simulink model "jiangyong_ZB2305010116"  (R2022b)
settings: Solver=VariableStepAuto  StartTime=0.0  StopTime=5  RelTol=1e-3
libraries: commdigbbndpm3 x4, commchan3 x2, commsink2 x2, commrandsrc3 x2
settings Model: Creator=JY  LastModifiedBy=JY

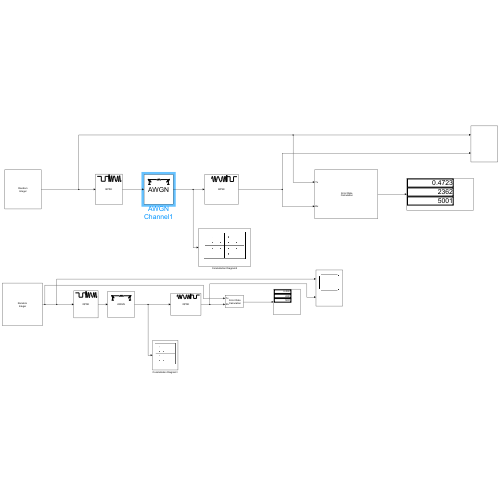
[thumbnail: Simulink's stored preview of the top-level diagram]
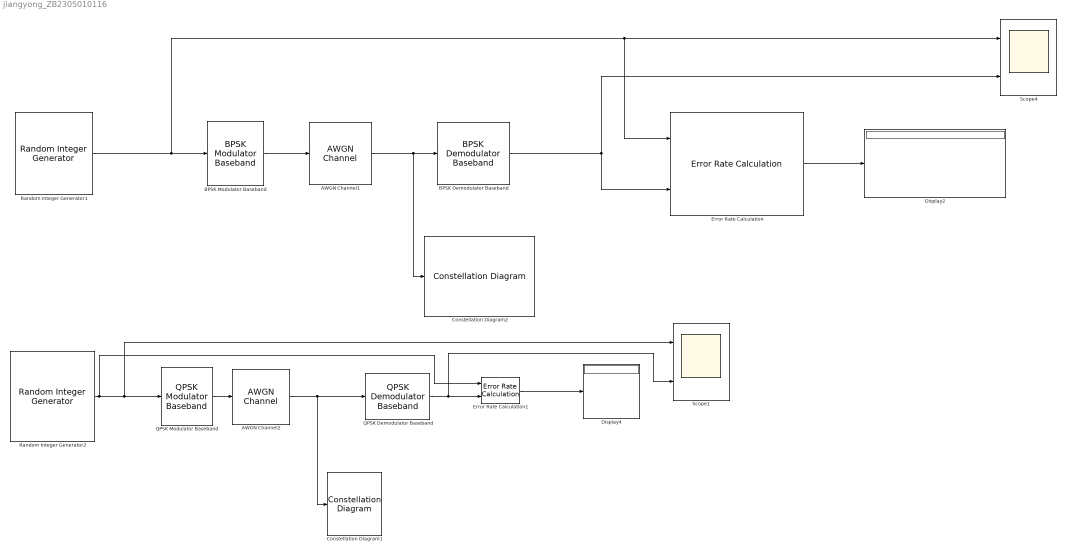
== system jiangyong_ZB2305010116 ==
  AWGN Channel1 : commchan3/AWGN Channel  InputProcessing=Columns as channels (frame based)  seed=67  noiseMode="Signal to noise ratio  (Eb/No)"  EbNodB=1  EsNodB=50  SNRdB=0  bitsPerSym=1  Ps=1  Tsym=1  variance=1
  AWGN Channel2 : commchan3/AWGN Channel  InputProcessing=Columns as channels (frame based)  seed=67  noiseMode="Signal to noise ratio  (Eb/No)"  EbNodB=9  EsNodB=10  SNRdB=0  bitsPerSym=1  Ps=2  Tsym=0.01  variance=1
  BPSK Demodulator Baseband : commdigbbndpm3/BPSK Demodulator Baseband  DecType=Hard decision  VarSource=Dialog  Variance=1  Ph=0  outDtype=Inherit via internal rule  derotateFactorWordLen=16  derotateFactorDataTypeStr=Inherit: Same word length as input  derotateFactorLastDataTypeStr=Inherit: Same word length as input
  BPSK Modulator Baseband : commdigbbndpm3/BPSK Modulator Baseband  Ph=0  outDtype=double  outWordLen=16  outUDDataType=sfix(16)  outFracLenMode=Best precision  outFracLen=15  outDataTypeStr=double  outLastDataTypeStr=double
  Constellation Diagram1 : ConstellationDiagram  WindowPosition=[707.000000,41.000000,600.000000,600.000000,]  ScopeFrameLocation=window  SymbolsToDisplaySource=Property  SymbolsToDisplay=1000  ReferenceConstellation=QPSK  XLimits=[-1.46,1.46]  YLimits=[-1.38,1.38]
  Constellation Diagram2 : ConstellationDiagram  WindowPosition=[-107.000000,-37.000000,1536.000000,793.000000,]  ScopeFrameLocation=window  SymbolsToDisplaySource=Property  SymbolsToDisplay=1000  ReferenceConstellation=BPSK  XLimits=[-8.74,7.74]  YLimits=[-7.14,8.15]
  Display2 : Display
  Display4 : Display
  Error Rate Calculation : commsink2/Error Rate Calculation  N=0  st_delay=0  cp_mode=Entire frame  subframe=[]  PMode=Port  WsName=ErrorVec  RsMode2=off  stop=off  numErr=100  maxBits=1e6
  Error Rate Calculation1 : commsink2/Error Rate Calculation  N=0  st_delay=0  cp_mode=Entire frame  subframe=[]  PMode=Port  WsName=ErrorVec  RsMode2=off  stop=off  numErr=100  maxBits=1e6
  QPSK Demodulator Baseband : commdigbbndpm3/QPSK Demodulator Baseband  OutType=Integer  DecType=Hard decision  VarSource=Dialog  Variance=1  Dec=Gray  Ph=2.35  outDtype1=Inherit via internal rule  outDtype2=Inherit via internal rule  derotateFactorWordLen=16  derotateFactorDataTypeStr=Inherit: Same word length as input  derotateFactorLastDataTypeStr=Inherit: Same word length as input
  QPSK Modulator Baseband : commdigbbndpm3/QPSK Modulator Baseband  InType=Integer  Enc=Gray  Ph=2.35  outDtype=double  outWordLen=16  outUDDataType=sfix(16)  outFracLenMode=Best precision  outFracLen=15  outDataTypeStr=double  outLastDataTypeStr=double
  Random Integer Generator1 : commrandsrc3/Random Integer Generator  SetSize=2  SeedSource=Parameter  Seed=37  SampleTime=1e-3  SamplesPerFrame=1  OutputDataType=double  SimulateUsing=Interpreted execution
  Random Integer Generator2 : commrandsrc3/Random Integer Generator  SetSize=4  SeedSource=Parameter  Seed=37  SampleTime=1e-3  SamplesPerFrame=1  OutputDataType=double  SimulateUsing=Interpreted execution
  Scope1 : Scope  NumInputPorts=2
  Scope4 : Scope  NumInputPorts=2
  wires:
  BPSK Demodulator Baseband/1 -> Error Rate Calculation/2, Scope4/2
  Random Integer Generator1/1 -> BPSK Modulator Baseband/1, Scope4/1, Error Rate Calculation/1
  BPSK Modulator Baseband/1 -> AWGN Channel1/1
  Error Rate Calculation/1 -> Display2/1
  Random Integer Generator2/1 -> Scope1/1, QPSK Modulator Baseband/1, Error Rate Calculation1/1
  QPSK Modulator Baseband/1 -> AWGN Channel2/1
  Error Rate Calculation1/1 -> Display4/1
  QPSK Demodulator Baseband/1 -> Scope1/2, Error Rate Calculation1/2
  AWGN Channel1/1 -> Constellation Diagram2/1, BPSK Demodulator Baseband/1
  AWGN Channel2/1 -> QPSK Demodulator Baseband/1, Constellation Diagram1/1
